simulink model "ss_kalmf"  (R2022b)
settings: Solver=ode5  StartTime=0.0  StopTime=30  FixedStep=.002  RelTol=1e-3
values from neighbouring files (symbols this model uses):
  a = 2    [RunMeFirst.m]
  A = exp(-a*Ts)    [RunMeFirst.m]    (also in linsys1.m = -a)
  B = 1    [RunMeFirst.m]    (also in linsys1.m = b)
  Bd = B * integral(@(tau) exp(Ts-tau),0,Ts)    [RunMeFirst.m]
  C = 1    [RunMeFirst.m]    (also in linsys1.m)
  D = 0    [RunMeFirst.m]    (also in linsys1.m)
  Qd = Q * G^2 * 1/(2*a) * (1 - exp(-2*a*Ts))    [RunMeFirst.m]
  R = .2    (= 0.2)    [RunMeFirst.m]    (also in linsys1.m = 0.5)
  Ts = .05    (= 0.05)    [RunMeFirst.m]    (also in linsys1.m = 0.1)
  x_0 = 2    [RunMeFirst.m]
  xe_0 = 3    [RunMeFirst.m]
undefined symbols (not defined in the file or in its folder): Discrete, K, Time
libraries: simulink x1, ctrlSharedLib x1
settings Model: Creator=hp_desktop  LastModifiedBy=hp_desktop

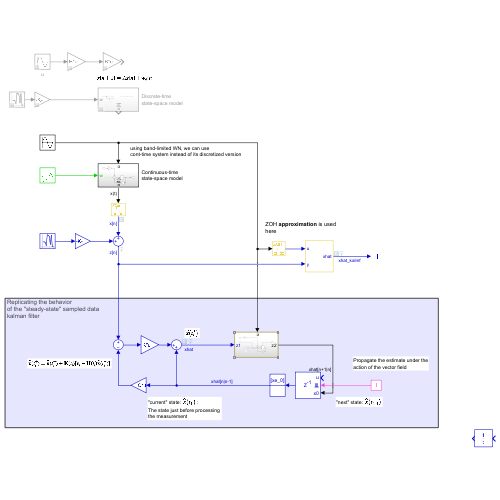
[thumbnail: Simulink's stored preview of the top-level diagram]
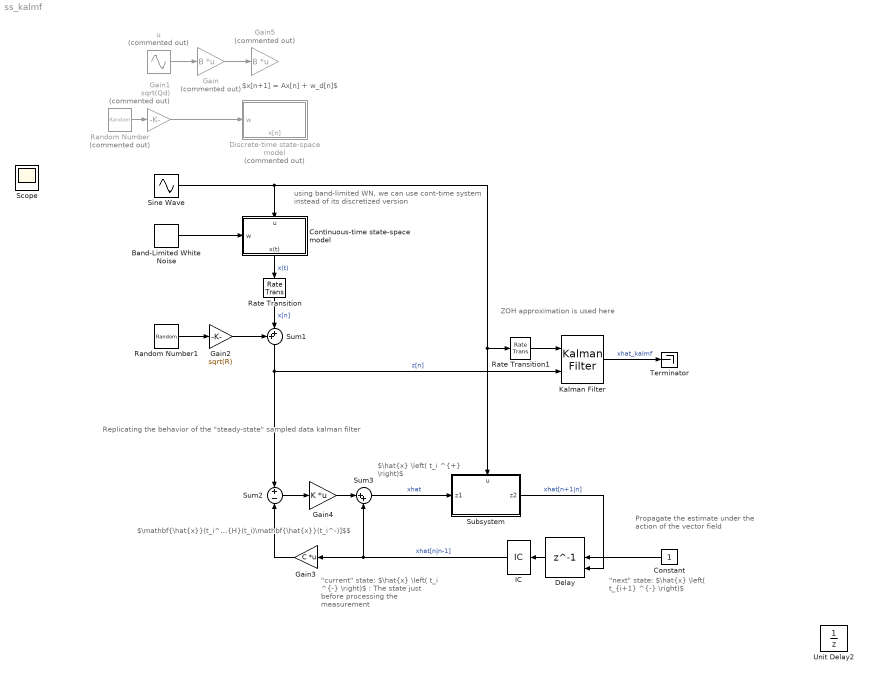
== system ss_kalmf ==
  note: using band-limited WN, we can use
      | cont-time system instead of its discretized version
  note: ZOH approximation is used
      | here
  note: Replicating the behavior
      | of the "steady-state" sampled data
      | kalman filter
  note: Propagate the estimate under the
      | action of the vector field
  note: $\mathbf{\hat{x}}(t_i^+)=\mathbf{\hat{x}}(t_i^-)+\mathbf{K}(t_i)[\mathbf{z}_i-\mathbf{H}(t_i)\mathbf{\hat{x}}(t_i^-)]$$
  note: "current" state: $\hat{x} \left( t_i ^{-} \right)$ :
      | The state just before processing
      | the measurement
  note: $x[n+1] = Ax[n] + w_d[n]$
  note: "next" state: $\hat{x} \left( t_{i+1} ^{-} \right)$
  note: $\hat{x} \left( t_i ^{+} \right)$
  Band-Limited White Noise : simulink/Sources/Band-Limited White Noise  Cov=Q  Ts=.01  seed=0
  Constant : Constant
  Continuous-time state-space model : Subsystem
      settings: PortSchema="{\"entries\":[{\"content\":{\"sides\":[{\"content\":{\"connectorIds\":[\"In1\"]},\"type\":\"ConnectorPlacement.EquallySpacedRectSide\",\"uuid\":\"03aefd50-9202-4ba5-8d59-8bb562bb4022\"},{\"content\":{\"connectorIds\":[],\"side\":\"RIGHT\"},\"type\":\"ConnectorPlacement.EquallySpacedRectSide\",\"uuid\":\"1686d747-63e6-444b-902a-9e9b0bc573f1\"},{\"content\":{\"connectorIds\":[\"In2\"],\"side\":\"TOP\"},\"type\":\"ConnectorPlacement.EquallySpacedRectSide\",\"uuid\":\"82334134-1918-4078-909d-97976d506e34\"},{\"content\":{\"connectorIds\":[\"Out1\"],\"side\":\"BOTTOM\"},\"type\":\"ConnectorPlacement.EquallySpacedRectSide\",\"uuid\":\"6a42f511-d3ae-4f43-bbaf-a2320965212b\"}]},\"type\":\"ConnectorPlacement.EquallySpacedConnector\",\"uuid\":\"1127eaf5-13bd-4ad9-99ec-3bc039f81ae3\"}],\"packageUris\":[\"http://schema.mathworks.com/mf0/Connector/R2020b\"],\"version\":\"1.0\"}"
  Delay : Delay  DelayLength=1  InitialConditionSource=Input port  ExternalReset=Level  SampleTime=Ts
      settings: InputPortMap=u0,r5,p4
  Discrete-time state-space model : Subsystem  Commented=on
      settings: PortSchema="{\"entries\":[{\"content\":{\"sides\":[{\"content\":{\"connectorIds\":[\"In1\"]},\"type\":\"ConnectorPlacement.EquallySpacedRectSide\",\"uuid\":\"03aefd50-9202-4ba5-8d59-8bb562bb4022\"},{\"content\":{\"connectorIds\":[],\"side\":\"RIGHT\"},\"type\":\"ConnectorPlacement.EquallySpacedRectSide\",\"uuid\":\"1686d747-63e6-444b-902a-9e9b0bc573f1\"},{\"content\":{\"connectorIds\":[],\"side\":\"TOP\"},\"type\":\"ConnectorPlacement.EquallySpacedRectSide\",\"uuid\":\"82334134-1918-4078-909d-97976d506e34\"},{\"content\":{\"connectorIds\":[\"Out1\"],\"side\":\"BOTTOM\"},\"type\":\"ConnectorPlacement.EquallySpacedRectSide\",\"uuid\":\"6a42f511-d3ae-4f43-bbaf-a2320965212b\"}]},\"type\":\"ConnectorPlacement.EquallySpacedConnector\",\"uuid\":\"1127eaf5-13bd-4ad9-99ec-3bc039f81ae3\"}],\"packageUris\":[\"http://schema.mathworks.com/mf0/Connector/R2020b\"],\"version\":\"1.0\"}"
  Gain : Gain  Commented=on  Gain=B  Multiplication=Matrix(K*u)
  Gain1 : Gain  Commented=on  Gain=sqrt(Qd)
  Gain2 : Gain  Gain=sqrt(R)
  Gain3 : Gain  Gain=C  Multiplication=Matrix(K*u)
  Gain4 : Gain  Gain=K  Multiplication=Matrix(K*u)
  Gain5 : Gain  Commented=on  Gain=B  Multiplication=Matrix(K*u)
  IC : InitialCondition  Value=xe_0
  Kalman Filter : ctrlSharedLib/Kalman Filter  TimeDomain=Discrete-Time  UseCurrentEstimator=on  ModelSource=Individual A, B, C, D matrices  ModelSourceVariable=ss(0.95,1,1,0,1)  A=A  B=Bd  C=C  D=D  NumberOfStates=1  NumberOfInputs=1  NumberOfOutputs=1  InitialEstimateSource=Dialog  X0=xe_0  P0=10  UseK=off  UseGH=off  NumberOfProcessNoiseInputs=1  G=1  TimeInvariantG=on  H=0  TimeInvariantH=on  Q=Qd  TimeInvariantQ=on  R=R  TimeInvariantR=on  N=0  TimeInvariantN=on  AddInputPort=on  AddEnablePort=off  OutputEstimatedY=off  OutputP=off  Ts=Ts
  Random Number : RandomNumber  Commented=on  SampleTime=Ts
  Random Number1 : RandomNumber  Seed=1503  SampleTime=Ts
  Rate Transition : RateTransition  OutPortSampleTime=Ts
  Rate Transition1 : RateTransition  OutPortSampleTime=Ts
  Sine Wave : Sin  Amplitude=.5  SampleTime=0
  Subsystem : Subsystem
      settings: PortSchema="{\"entries\":[{\"content\":{\"sides\":[{\"content\":{\"connectorIds\":[\"In1\"]},\"type\":\"ConnectorPlacement.EquallySpacedRectSide\",\"uuid\":\"5747362d-5452-450f-891f-9375624e3e6b\"},{\"content\":{\"connectorIds\":[\"Out1\"],\"side\":\"RIGHT\"},\"type\":\"ConnectorPlacement.EquallySpacedRectSide\",\"uuid\":\"0cdea8a7-8f51-46ce-9c0a-38e1d0ef94d4\"},{\"content\":{\"connectorIds\":[\"In2\"],\"side\":\"TOP\"},\"type\":\"ConnectorPlacement.EquallySpacedRectSide\",\"uuid\":\"b6652ee9-d7b3-4726-a52a-b0571aa84108\"}]},\"type\":\"ConnectorPlacement.EquallySpacedConnector\",\"uuid\":\"86b3c6e5-6cb8-4d7e-97aa-66bd2052fcbe\"}],\"packageUris\":[\"http://schema.mathworks.com/mf0/Connector/R2020b\"],\"version\":\"1.0\"}"
  Sum1 : Sum  Inputs=++|
  Sum2 : Sum  Inputs=+-
  Sum3 : Sum  Inputs=|++
  Terminator : Terminator
  Unit Delay2 : UnitDelay  InitialCondition=xe_0  SampleTime=Ts  HasFrameUpgradeWarning=on
  u : Sin  Commented=on  Amplitude=.5  SampleTime=0
  Scope : Scope
  wires:
  Random Number/1 -> Gain1/1
  Random Number1/1 -> Gain2/1
  Gain2/1 -> Sum1/1
  Sum1/1 -> Sum2/1, Kalman Filter/2  "z[n]"
  IC/1 -> Sum3/2, Gain3/1  "xhat[n|n-1]"
  Gain3/1 -> Sum2/2
  Sum2/1 -> Gain4/1
  Gain4/1 -> Sum3/1
  Rate Transition1/1 -> Kalman Filter/1
  Kalman Filter/1 -> Terminator/1  "xhat_kalmf"
  Gain1/1 -> Discrete-time state-space model/1(w)
  Sum3/1 -> Subsystem/1(z1)  "xhat"
  Subsystem/1(z2) -> Delay/3  "xhat[n+1|n]"
  Constant/1 -> Delay/2
  Delay/1 -> IC/1
  u/1 -> Gain/1
  Gain/1 -> Gain5/1
  Band-Limited White Noise/1 -> Continuous-time state-space model/1(w)
  Continuous-time state-space model/1(x(t)) -> Rate Transition/1  "x(t)"
  Rate Transition/1 -> Sum1/2  "x[n]"
  Sine Wave/1 -> Rate Transition1/1, Subsystem/2(u), Continuous-time state-space model/2(u)

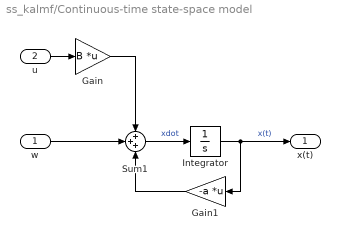
== system ss_kalmf/Continuous-time state-space model ==
  w : Inport
  u : Inport  Port=2
  Gain : Gain  Gain=B  Multiplication=Matrix(K*u)
  Gain1 : Gain  Gain=-a  Multiplication=Matrix(K*u)
  Integrator : Integrator  InitialCondition=x_0
  Sum1 : Sum  Inputs=+++
  x(t) : Outport
  wires:
  Integrator/1 -> x(t)/1, Gain1/1  "x(t)"
  Sum1/1 -> Integrator/1  "xdot"
  Gain1/1 -> Sum1/3
  w/1 -> Sum1/2
  Gain/1 -> Sum1/1
  u/1 -> Gain/1

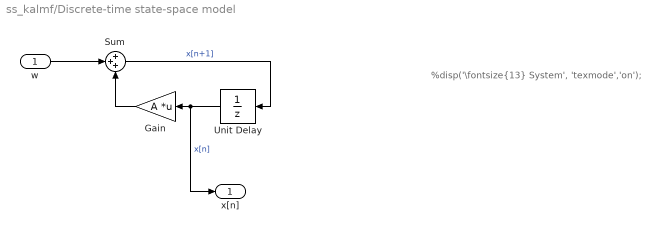
== system ss_kalmf/Discrete-time state-space model ==
  note: %disp('\fontsize{13} System', 'texmode','on');
  w : Inport
  Gain : Gain  Gain=A  Multiplication=Matrix(K*u)
  Sum : Sum  Inputs=+++
  Unit Delay : UnitDelay  InitialCondition=x_0  SampleTime=Ts  HasFrameUpgradeWarning=on
  x[n] : Outport
  wires:
  Unit Delay/1 -> x[n]/1, Gain/1  "x[n]"
  Gain/1 -> Sum/3
  Sum/1 -> Unit Delay/1  "x[n+1]"
  w/1 -> Sum/2

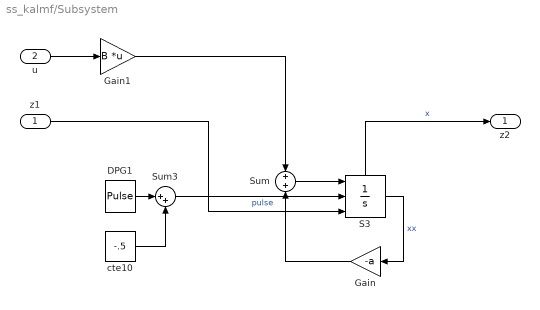
== system ss_kalmf/Subsystem ==
  z1 : Inport
  u : Inport  Port=2
  DPG1 : DiscretePulseGenerator  SampleTime=Ts
  Gain : Gain  Gain=-a
  Gain1 : Gain  Gain=B  Multiplication=Matrix(K*u)
  S3 : Integrator  ExternalReset=either  InitialConditionSource=external  ShowStatePort=on
  Sum : Sum
  Sum3 : Sum  Inputs=|++
  cte10 : Constant  Value=-.5
  z2 : Outport
  wires:
  cte10/1 -> Sum3/2
  Sum3/1 -> S3/2  "pulse"
  DPG1/1 -> Sum3/1
  S3/1 -> Gain/1  "xx"
  z1/1 -> S3/3
  S3/State -> z2/1  "x"
  Gain1/1 -> Sum/1
  u/1 -> Gain1/1
  Gain/1 -> Sum/2
  Sum/1 -> S3/1
